simulink model "Regulation_with_aging"  (R2018a)
settings: Solver=VariableStepAuto  StartTime=0.0  StopTime=10.0  RelTol=1e-3
values from neighbouring files (symbols this model uses):
  A = double(A)    [Linearization.m]    (also in findK_emtiazi.m = [1 2 0; 0 -1 3; 0 1 -1])
  B = double(B)    [Linearization.m]
  C = [1 0 0 0 ; 0 1 0 0 ]    [Linearization.m]    (also in findK_emtiazi.m = [0 1 0])
  Gcl = inv(C*inv(-A+B*k)*B)    [Linearization.m]
  k = place(A,B,pc)    [Linearization.m]
settings Model: Creator=YaCn  LastModifiedBy=YaCn

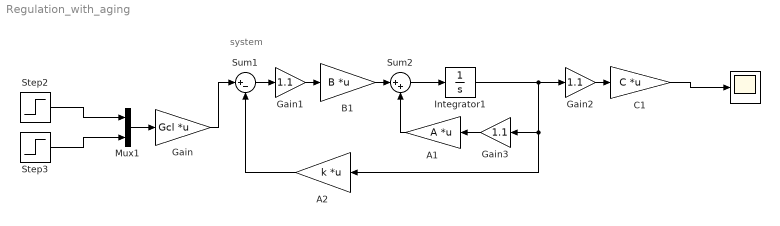
== system Regulation_with_aging ==
  note: system
  " " : Scope
  A1 : Gain  Gain=A  Multiplication=Matrix(K*u) (u vector)
  A2 : Gain  Gain=k  Multiplication=Matrix(K*u) (u vector)
  B1 : Gain  Gain=B  Multiplication=Matrix(K*u) (u vector)
  C1 : Gain  Gain=C  Multiplication=Matrix(K*u) (u vector)
  Gain : Gain  Gain=Gcl  Multiplication=Matrix(K*u) (u vector)
  Gain1 : Gain  Gain=1.1
  Gain2 : Gain  Gain=1.1
  Gain3 : Gain  Gain=1.1
  Integrator1 : Integrator
  Mux1 : Mux  Inputs=2
  Step2 : Step  Time=0  SampleTime=0.0001
  Step3 : Step  Time=0  After=1.2  SampleTime=0.001
  Sum1 : Sum  Inputs=|+-
  Sum2 : Sum  Inputs=|++
  wires:
  Gain/1 -> Sum1/1
  A2/1 -> Sum1/2
  Mux1/1 -> Gain/1
  Sum2/1 -> Integrator1/1
  Integrator1/1 -> Gain2/1, Gain3/1, A2/1
  B1/1 -> Sum2/1
  Step2/1 -> Mux1/1
  Step3/1 -> Mux1/2
  Sum1/1 -> Gain1/1
  Gain1/1 -> B1/1
  C1/1 -> " "/1
  Gain3/1 -> A1/1
  A1/1 -> Sum2/2
  Gain2/1 -> C1/1
